simulink model "sixth_10_03_25"  (R2024b)
settings: Solver=VariableStepAuto  StartTime=0.0  StopTime=inf  MaxStep=1e-5  RelTol=1e-3
undefined symbols (not defined in the file): fsw, l, r
libraries: simulink x3
settings Model: Creator=claudio.rossi  LastModifiedBy=Franco
settings OptimizationCC: ReuseModelBlockBuffer=off
settings RTWCC: GPUComputeCapability=3.5

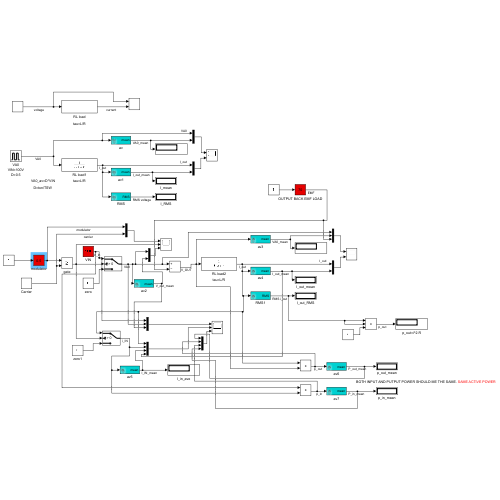
[thumbnail: Simulink's stored preview of the top-level diagram]
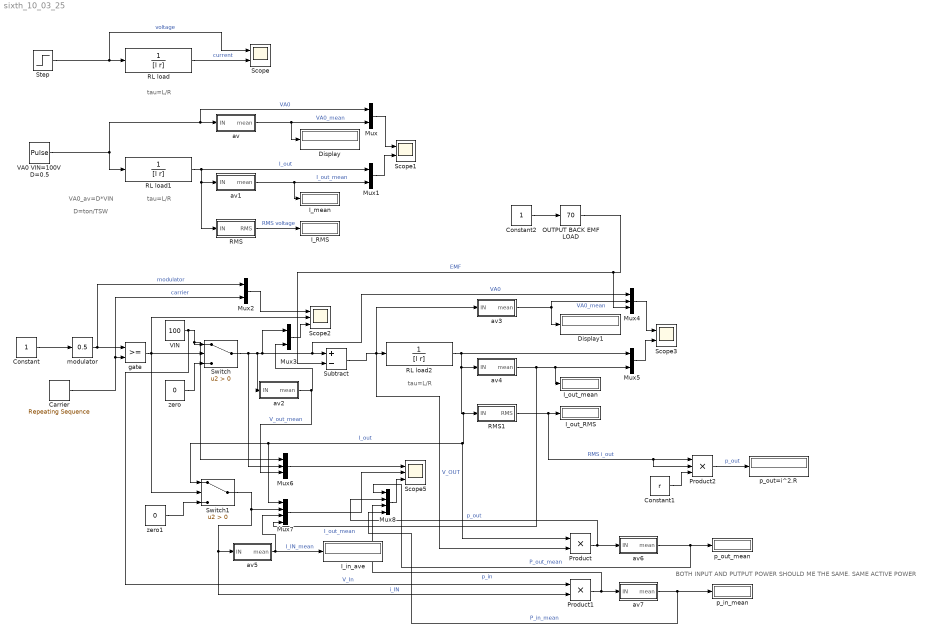
== system sixth_10_03_25 ==
  note: BOTH INPUT AND PUTPUT POWER SHOULD ME THE SAME. SAME ACTIVE POWER
  note: VA0_av=D*VIN
  note: D=ton/TSW
  note: tau=L/R
  note: tau=L/R
  note: tau=L/R
  "Carrier " : simulink/Sources/Repeating Sequence  rep_seq_t=[0 0.5/fsw 1/fsw]  rep_seq_y=[0 1 0 ]
  Constant : Constant
  Constant1 : Constant  Value=r
  Constant2 : Constant
  Display : Display
  Display1 : Display
  I_RMS : Display
  I_in_ave : Display
  I_mean : Display
  I_out_RMS : Display
  I_out_mean : Display
  Mux{,1..3,5} (5 alike) : Mux  Inputs=2
  Mux4 : Mux  Inputs=3
  Mux6 : Mux  Inputs=3
  Mux7 : Mux
  Mux8 : Mux
  OUTPUT BACK EMF LOAD : simulink/Math Operations/Slider Gain  gain=70  low=0  high=100
  Product : Product
  Product1 : Product
  Product2 : Product  Inputs=3
  RL load : TransferFcn  Denominator=[l r]
  RL load1 : TransferFcn  Denominator=[l r]
  RL load2 : TransferFcn  Denominator=[l r]
  RMS : Subsystem  mask{period=1/fsw}
      mask prompts: period "period [s]"
      mask DialogControl DescTextVar Prompt: calculates the RMS of a periodic function with period specified here
  RMS1 : Subsystem  mask{period=1/fsw}
      mask prompts: period "period [s]"
      mask DialogControl DescTextVar Prompt: calculates the RMS of a periodic function with period specified here
  Scope : Scope  NumInputPorts=2
  Scope1 : Scope  NumInputPorts=2
  Scope2 : Scope  NumInputPorts=3
  Scope3 : Scope  NumInputPorts=2
  Scope5 : Scope  NumInputPorts=3
  Step : Step  After=100  SampleTime=0
  Subtract : Sum  Inputs=+-
  Switch : Switch  Criteria=u2 > Threshold  SaturateOnIntegerOverflow=off  InputSameDT=off
  Switch1 : Switch  Criteria=u2 > Threshold  SaturateOnIntegerOverflow=off  InputSameDT=off
  VA0 VIN=100V D=0.5 : DiscretePulseGenerator  PulseType=Time based  Amplitude=100  Period=1/fsw  PulseWidth=50
  VIN : Constant  Value=100
  av : Subsystem  mask{period=1/fsw}
      mask prompts: period "period [s]"
      mask DialogControl DescTextVar Prompt: calculate the averge over period
      mask DialogControl text Prompt: test
  av1 : Subsystem  mask{period=1/fsw}
      mask prompts: period "period [s]"
      mask DialogControl DescTextVar Prompt: calculate the averge over period
      mask DialogControl text Prompt: test
  av2 : Subsystem  mask{period=1/fsw}
      mask prompts: period "period [s]"
      mask DialogControl DescTextVar Prompt: calculate the averge over period
      mask DialogControl text Prompt: test
  av3 : Subsystem  mask{period=1/fsw}
      mask prompts: period "period [s]"
      mask DialogControl DescTextVar Prompt: calculate the averge over period
      mask DialogControl text Prompt: test
  av4 : Subsystem  mask{period=1/fsw}
      mask prompts: period "period [s]"
      mask DialogControl DescTextVar Prompt: calculate the averge over period
      mask DialogControl text Prompt: test
  av5 : Subsystem  mask{period=1/fsw}
      mask prompts: period "period [s]"
      mask DialogControl DescTextVar Prompt: calculate the averge over period
      mask DialogControl text Prompt: test
  av6 : Subsystem  mask{period=1/fsw}
      mask prompts: period "period [s]"
      mask DialogControl DescTextVar Prompt: calculate the averge over period
      mask DialogControl text Prompt: test
  av7 : Subsystem  mask{period=1/fsw}
      mask prompts: period "period [s]"
      mask DialogControl DescTextVar Prompt: calculate the averge over period
      mask DialogControl text Prompt: test
  gate : RelationalOperator  OutDataTypeStr=boolean  RndMeth=Simplest  InputSameDT=off
  modulator : simulink/Math Operations/Slider Gain  gain=0.5  low=0  high=1
  p_in_mean : Display
  p_out=i^2.R : Display
  p_out_mean : Display
  zero : Constant  Value=0
  zero1 : Constant  Value=0
  wires:
  Step/1 -> Scope/1, RL load/1  "voltage"
  RL load/1 -> Scope/2  "current"
  VA0 VIN=100V D=0.5/1 -> RL load1/1, Mux/1, av/1(IN)  "VA0"
  av/1(mean) -> Display/1, Mux/2  "VA0_mean"
  Mux/1 -> Scope1/1
  av1/1(mean) -> I_mean/1, Mux1/2  "I_out_mean"
  Mux1/1 -> Scope1/2
  RL load1/1 -> Mux1/1, RMS/1(IN), av1/1(IN)  "I_out"
  RMS/1(RMS) -> I_RMS/1  "RMS voltage"
  "Carrier "/1 -> Mux2/2, gate/2  "carrier"
  Constant/1 -> modulator/1
  modulator/1 -> Mux2/1, gate/1  "modulator"
  gate/1 -> Switch1/2, Switch/2, Scope2/2
  VIN/1 -> Mux6/1, Switch/1, Product1/1  "V_In"
  zero/1 -> Switch/3
  Mux2/1 -> Scope2/1
  Mux3/1 -> Scope2/3
  Switch/1 -> Mux6/2, av2/1(IN), Mux4/1, Subtract/1, Mux3/1  "VA0"
  av2/1(mean) -> Mux6/3, Mux3/2  "V_out_mean"
  RMS1/1(RMS) -> Product2/2, Product2/1, I_out_RMS/1  "RMS i_out"
  RL load2/1 -> av4/1(IN), Product/1, Mux7/1, Switch1/1, RMS1/1(IN), Mux5/1  "I_out"
  Mux5/1 -> Scope3/2
  av4/1(mean) -> Mux7/4, Mux5/2, I_out_mean/1  "I_out_mean"
  Mux4/1 -> Scope3/1
  av3/1(mean) -> Mux4/2, Display1/1  "VA0_mean"
  zero1/1 -> Switch1/3
  Mux6/1 -> Scope5/1
  Switch1/1 -> Product1/2, av5/1(IN), Mux7/2  "i_IN"
  Mux7/1 -> Scope5/2
  av5/1(mean) -> Mux7/3, I_in_ave/1  "I_IN_mean"
  Product/1 -> Mux8/2, av6/1(IN)  "p_out"
  av6/1(mean) -> Mux8/1, p_out_mean/1  "P_out_mean"
  av7/1(mean) -> Mux8/4, p_in_mean/1  "P_in_mean"
  Product1/1 -> Mux8/3, av7/1(IN)  "p_in"
  Constant1/1 -> Product2/3
  Product2/1 -> p_out=i^2.R/1  "p_out"
  Mux8/1 -> Scope5/3
  Constant2/1 -> OUTPUT BACK EMF LOAD/1
  Subtract/1 -> Product/2, av3/1(IN), RL load2/1  "V_OUT"
  OUTPUT BACK EMF LOAD/1 -> Mux4/3, Subtract/2  "EMF"

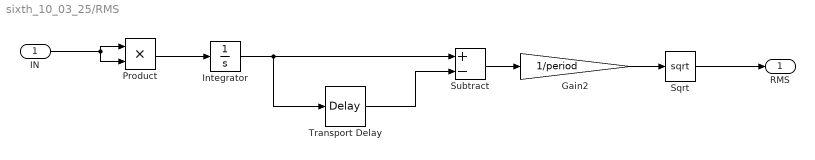
== system sixth_10_03_25/RMS ==
  IN : Inport
  Gain2 : Gain  Gain=1/period
  Integrator : Integrator
  Product : Product
  Sqrt : Sqrt
  Subtract : Sum  Inputs=+-
  Transport Delay : TransportDelay  DelayTime=period
  RMS : Outport
  wires:
  Sqrt/1 -> RMS/1
  Gain2/1 -> Sqrt/1
  Product/1 -> Integrator/1
  IN/1 -> Product/2, Product/1
  Integrator/1 -> Transport Delay/1, Subtract/1
  Subtract/1 -> Gain2/1
  Transport Delay/1 -> Subtract/2

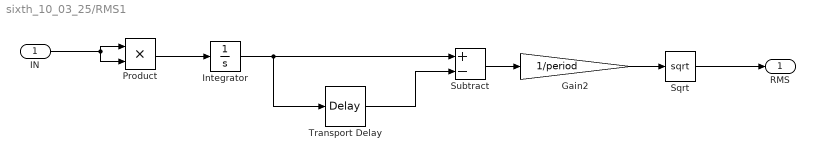
== system sixth_10_03_25/RMS1 ==
  IN : Inport
  Gain2 : Gain  Gain=1/period
  Integrator : Integrator
  Product : Product
  Sqrt : Sqrt
  Subtract : Sum  Inputs=+-
  Transport Delay : TransportDelay  DelayTime=period
  RMS : Outport
  wires:
  Transport Delay/1 -> Subtract/2
  Subtract/1 -> Gain2/1
  Integrator/1 -> Subtract/1, Transport Delay/1
  IN/1 -> Product/1, Product/2
  Product/1 -> Integrator/1
  Gain2/1 -> Sqrt/1
  Sqrt/1 -> RMS/1

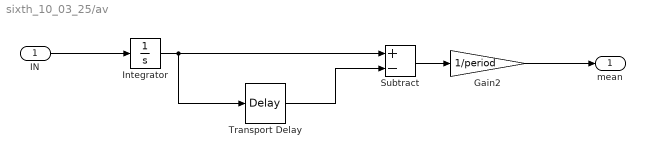
== system sixth_10_03_25/av ==
  IN : Inport
  Gain2 : Gain  Gain=1/period
  Integrator : Integrator
  Subtract : Sum  Inputs=+-
  Transport Delay : TransportDelay  DelayTime=period
  mean : Outport
  wires:
  Integrator/1 -> Transport Delay/1, Subtract/1
  Gain2/1 -> mean/1
  Subtract/1 -> Gain2/1
  Transport Delay/1 -> Subtract/2
  IN/1 -> Integrator/1

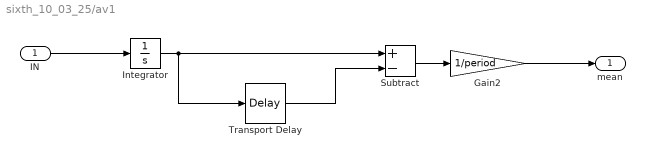
== system sixth_10_03_25/av1 ==
  IN : Inport
  Gain2 : Gain  Gain=1/period
  Integrator : Integrator
  Subtract : Sum  Inputs=+-
  Transport Delay : TransportDelay  DelayTime=period
  mean : Outport
  wires:
  IN/1 -> Integrator/1
  Transport Delay/1 -> Subtract/2
  Subtract/1 -> Gain2/1
  Gain2/1 -> mean/1
  Integrator/1 -> Subtract/1, Transport Delay/1

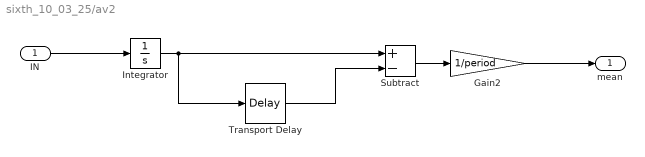
== system sixth_10_03_25/av2 ==
  IN : Inport
  Gain2 : Gain  Gain=1/period
  Integrator : Integrator
  Subtract : Sum  Inputs=+-
  Transport Delay : TransportDelay  DelayTime=period
  mean : Outport
  wires:
  Integrator/1 -> Transport Delay/1, Subtract/1
  Gain2/1 -> mean/1
  Subtract/1 -> Gain2/1
  Transport Delay/1 -> Subtract/2
  IN/1 -> Integrator/1

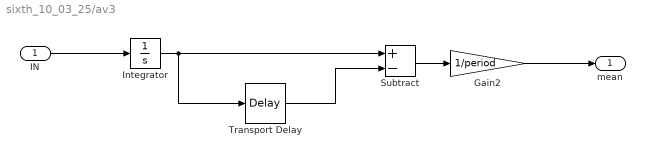
== system sixth_10_03_25/av3 ==
  IN : Inport
  Gain2 : Gain  Gain=1/period
  Integrator : Integrator
  Subtract : Sum  Inputs=+-
  Transport Delay : TransportDelay  DelayTime=period
  mean : Outport
  wires:
  IN/1 -> Integrator/1
  Transport Delay/1 -> Subtract/2
  Subtract/1 -> Gain2/1
  Gain2/1 -> mean/1
  Integrator/1 -> Subtract/1, Transport Delay/1

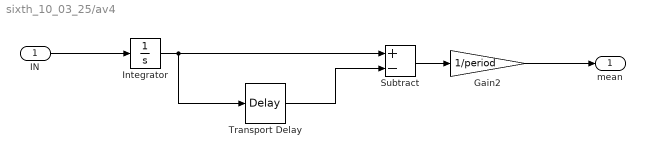
== system sixth_10_03_25/av4 ==
  IN : Inport
  Gain2 : Gain  Gain=1/period
  Integrator : Integrator
  Subtract : Sum  Inputs=+-
  Transport Delay : TransportDelay  DelayTime=period
  mean : Outport
  wires:
  Integrator/1 -> Transport Delay/1, Subtract/1
  Gain2/1 -> mean/1
  Subtract/1 -> Gain2/1
  Transport Delay/1 -> Subtract/2
  IN/1 -> Integrator/1

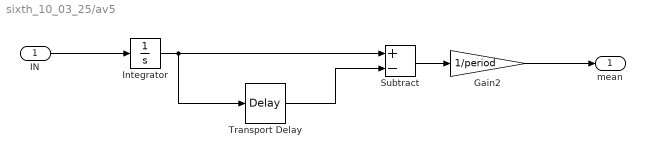
== system sixth_10_03_25/av5 ==
  IN : Inport
  Gain2 : Gain  Gain=1/period
  Integrator : Integrator
  Subtract : Sum  Inputs=+-
  Transport Delay : TransportDelay  DelayTime=period
  mean : Outport
  wires:
  IN/1 -> Integrator/1
  Transport Delay/1 -> Subtract/2
  Subtract/1 -> Gain2/1
  Gain2/1 -> mean/1
  Integrator/1 -> Subtract/1, Transport Delay/1

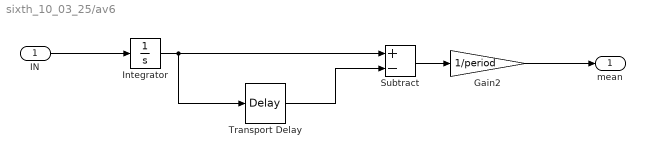
== system sixth_10_03_25/av6 ==
  IN : Inport
  Gain2 : Gain  Gain=1/period
  Integrator : Integrator
  Subtract : Sum  Inputs=+-
  Transport Delay : TransportDelay  DelayTime=period
  mean : Outport
  wires:
  IN/1 -> Integrator/1
  Transport Delay/1 -> Subtract/2
  Subtract/1 -> Gain2/1
  Gain2/1 -> mean/1
  Integrator/1 -> Subtract/1, Transport Delay/1

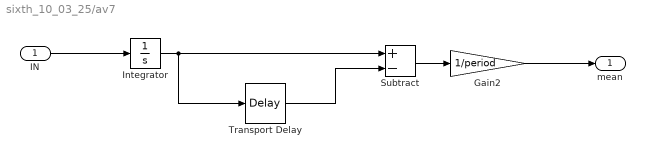
== system sixth_10_03_25/av7 ==
  IN : Inport
  Gain2 : Gain  Gain=1/period
  Integrator : Integrator
  Subtract : Sum  Inputs=+-
  Transport Delay : TransportDelay  DelayTime=period
  mean : Outport
  wires:
  Integrator/1 -> Transport Delay/1, Subtract/1
  Gain2/1 -> mean/1
  Subtract/1 -> Gain2/1
  Transport Delay/1 -> Subtract/2
  IN/1 -> Integrator/1
